simulink model "gatorKator_spectrum_visualization_with_frame_counter"  (Simulink 7.7)
settings: Solver=FixedStepDiscrete  StartTime=21e-3  StopTime=60  RelTol=1e-3
undefined symbols (not defined in the file or in its folder): jet
libraries: dspsnks4 x3, simulink x1, dspswit3 x1, dspsrcs4 x1, dspindex x1, dspspect3 x1, dspmtrx3 x1, dspmathops x1
settings Model: Creator=staticd  LastModifiedBy=staticd

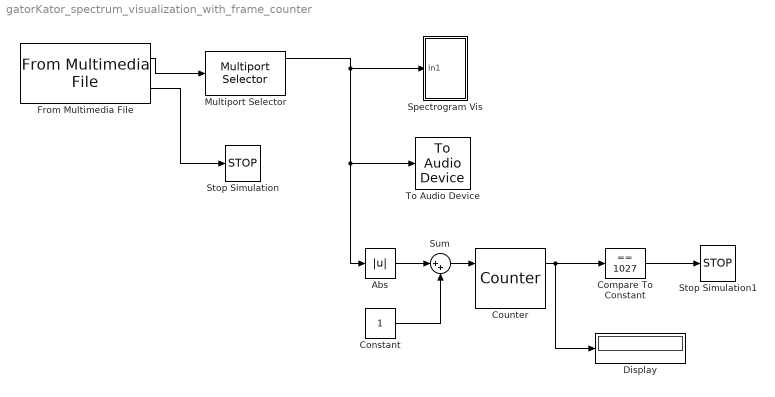
== system gatorKator_spectrum_visualization_with_frame_counter ==
  Abs : Abs
  Compare To Constant : simulink/Logic and Bit Operations/Compare To Constant  SystemSampleTime=-1  relop===  const=1027  LogicOutDataTypeMode=boolean
  Constant : Constant
  Counter : dspswit3/Counter  Direction=Up  CountEvent=Non-zero sample  CounterSize=User defined  MaxCount=1e6  InitialCount=0  Output=Count and Hit  HitValue=32  ResetInput=on  SamplesPerFrame=1  Ts=1  CntDtype=double  HitDtype=Logical
  Display : Display
  From Multimedia File : dspsrcs4/From Multimedia File  inputFilename=C:\Users\staticd\Documents\COLLEGE\EEL 4935 DSP_FPGA\project\26alligator1bellow.mp3  loop=on  numPlays=inf  outputStreams=Audio only  videoDataType=single  audioDataType=double  inheritSampleTime=on  userDefinedSampleTime=1/30  noAudioOutput=off  isIntensityVideo=off  fourcc=RGB  colorVideoFormat=Separate color signals  outputEOF=on  dataOrg=Column-major  audioFrameSize=1024  computeAudioFrameSize=off
  Multiport Selector : dspindex/Multiport Selector  rowsOrCols=Columns  idxCellArray={ 4, [1:2 5], [7; 8], 10:-1:6 }  idxErrMode=Clip Index
  Spectrogram Vis : Subsystem
  Stop Simulation : Stop
  Stop Simulation1 : Stop
  Sum : Sum  Inputs=|++
  To Audio Device : dspsnks4/To Audio Device  deviceName=Default  inheritSampleRate=on  sampleRate=44100  deviceDatatype=Determine from input data type  autoBufferSize=on  bufferSize=4096  queueDuration=1.0
  wires:
  From Multimedia File/1 -> Multiport Selector/1
  Multiport Selector/1 -> Spectrogram Vis/1(In1), To Audio Device/1, Abs/1
  From Multimedia File/2 -> Stop Simulation/1
  Counter/1 -> Compare To Constant/1, Display/1
  Compare To Constant/1 -> Stop Simulation1/1
  Abs/1 -> Sum/1
  Constant/1 -> Sum/2
  Sum/1 -> Counter/1

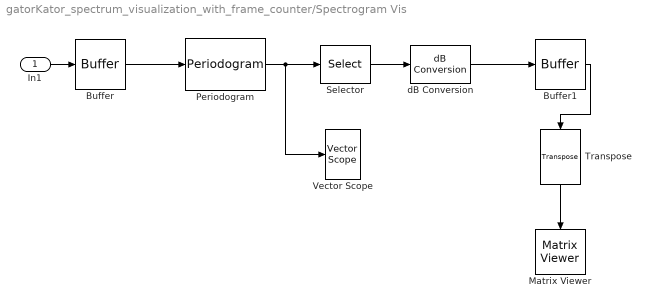
== system gatorKator_spectrum_visualization_with_frame_counter/Spectrogram Vis ==
  In1 : Inport
  Buffer : Buffer  N=256  TreatMby1Signals=One channel
  Buffer1 : Buffer  V=60  ic=-1
  Matrix Viewer : dspsnks4/Matrix Viewer  ImageParams=off  CMapStr=jet(256)  AxisColorbar=on  AxisParams=off  AxisOrigin=Lower left corner  XLabel=Time Index  YLabel=Frequency Index  ZLabel=dB Magnitude  FigPos=[50 530 1300 320]  AxisZoom=off
      settings: YMin=-80  YMax=10
  Periodogram : dspspect3/Periodogram  SystemSampleTime=-1  measurement=Power spectral density  wintype=Hamming  Rs=50  beta=5  winsamp=Periodic  inheritFFT=on  fftsize=256  navg=1  inheritTs=on  Ts=1
  Selector : Selector  InputPortWidth=256  IndexOptions=Index vector (dialog)  Indices=[1:128]  OutputSizes=1
  Transpose : dspmtrx3/Transpose  SystemSampleTime=-1  Hermitian=off  overflowFlag=off
  Vector Scope : dspsnks4/Vector Scope  ScopeProperties=on  Domain=Frequency  HorizSpan=1  DisplayProperties=off  AxisGrid=on  Memory=off  FrameNumber=on  AxisLegend=off  AxisZoom=off  OpenScopeAtSimStart=on  OpenScopeImmediately=off  FigPos=[50 110 1300 320]  AxisProperties=off  XUnits=Hertz  XRange=[0...Fs/2]  InheritXIncr=on  XIncr=1  XLabel=Time  XLimit=User-defined  XMin=0  XMax=3.5e3  XStart=0  YUnits=dB  YLabel=Magnitude, dB  LineProperties=off  XAxisParamsVer=6.9
      settings: YMin=-80  YMax=10
  dB Conversion : dspmathops/dB Conversion  SystemSampleTime=-1  dBtype=dB  intype=Power  R=1  fuzz=on
  wires:
  In1/1 -> Buffer/1
  Transpose/1 -> Matrix Viewer/1
  Buffer1/1 -> Transpose/1
  dB Conversion/1 -> Buffer1/1
  Selector/1 -> dB Conversion/1
  Periodogram/1 -> Vector Scope/1, Selector/1
  Buffer/1 -> Periodogram/1
